simulink model "lab3_ss_srl"  (R2024b)
settings: Solver=ode45  StartTime=0.0  StopTime=sIn.simulation_time  RelTol=1e-3
undefined symbols (not defined in the file or in its folder): daq, drv, feedback, filt, gbox, mld, mot, rads2rpm, sens, sIn
settings Model: Creator=pries  LastModifiedBy=Nihal
settings DataIOCC: SaveOutput=off  SaveTime=off  ReturnWorkspaceOutputs=off

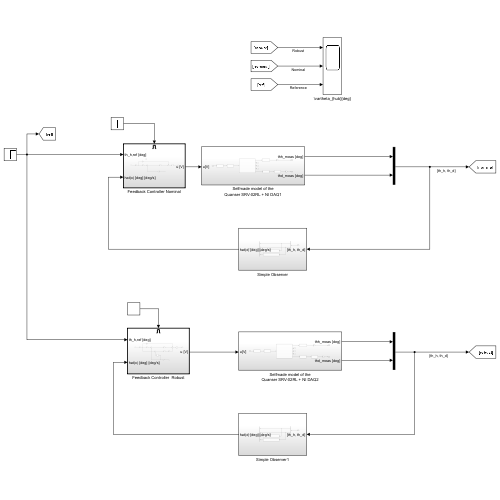
[thumbnail: Simulink's stored preview of the top-level diagram]
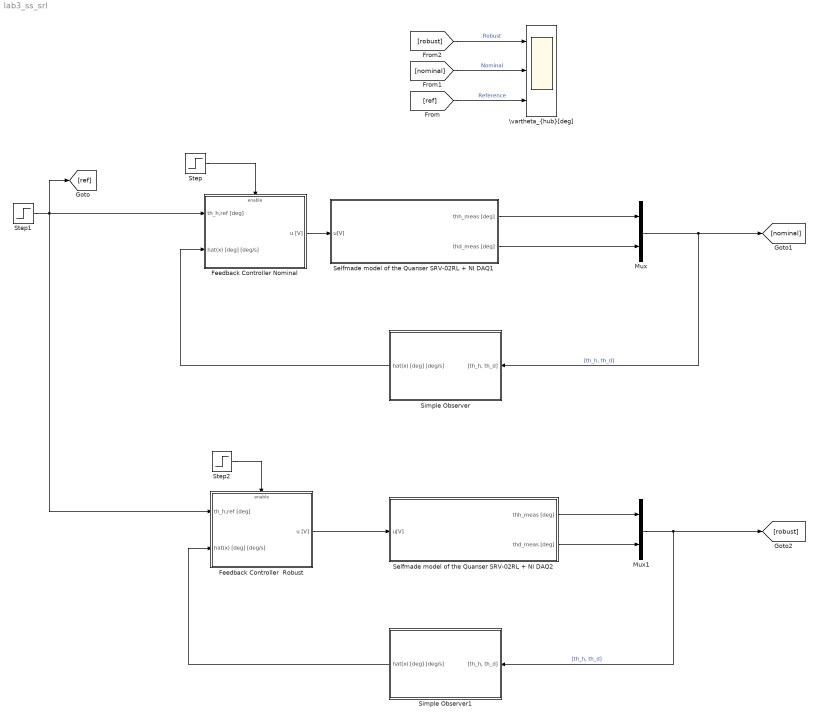
== system lab3_ss_srl ==
  Feedback Controller  Robust : Subsystem
  Feedback Controller Nominal : Subsystem
  Mux : Mux  Inputs=2
  Mux1 : Mux  Inputs=2
  Selfmade model of the Quanser SRV-02RL + NI DAQ1 : Subsystem
  Selfmade model of the Quanser SRV-02RL + NI DAQ2 : Subsystem
  Simple Observer : Subsystem
  Simple Observer1 : Subsystem
  Step : Step  Time=sIn.t1  SampleTime=0
  Step1 : Step  Time=sIn.t1  After=sIn.position  SampleTime=0
  Step2 : Step  Time=sIn.t1  SampleTime=0
  "\\vartheta_{hub}[deg]" : Scope  NumInputPorts=3
  wires:
  Mux/1 -> [nominal], Simple Observer/1("[th_h, th_d]")  "[th_h, th_d]"
  Simple Observer/1(hat(x) [deg] [deg/s]) -> Feedback Controller Nominal/2(hat(x) [deg] [deg/s])
  Step/1 -> Feedback Controller Nominal/Enable
  Step1/1 -> Feedback Controller  Robust/1(th_h,ref [deg]), Feedback Controller Nominal/1(th_h,ref [deg]), [ref]
  Simple Observer1/1(hat(x) [deg] [deg/s]) -> Feedback Controller  Robust/2(hat(x) [deg] [deg/s])
  [robust] -> "\\vartheta_{hub}[deg]"/1  "Robust"
  [nominal] -> "\\vartheta_{hub}[deg]"/2  "Nominal"
  [ref] -> "\\vartheta_{hub}[deg]"/3  "Reference"
  Feedback Controller  Robust/1(u [V]) -> Selfmade model of the Quanser SRV-02RL + NI DAQ2/1(u[V])
  Step2/1 -> Feedback Controller  Robust/Enable
  Feedback Controller Nominal/1(u [V]) -> Selfmade model of the Quanser SRV-02RL + NI DAQ1/1(u[V])
  Selfmade model of the Quanser SRV-02RL + NI DAQ1/1(thh_meas [deg]) -> Mux/1
  Selfmade model of the Quanser SRV-02RL + NI DAQ1/2(thd_meas [deg]) -> Mux/2
  Selfmade model of the Quanser SRV-02RL + NI DAQ2/1(thh_meas [deg]) -> Mux1/1
  Selfmade model of the Quanser SRV-02RL + NI DAQ2/2(thd_meas [deg]) -> Mux1/2
  Mux1/1 -> [robust], Simple Observer1/1("[th_h, th_d]")  "[th_h, th_d]"

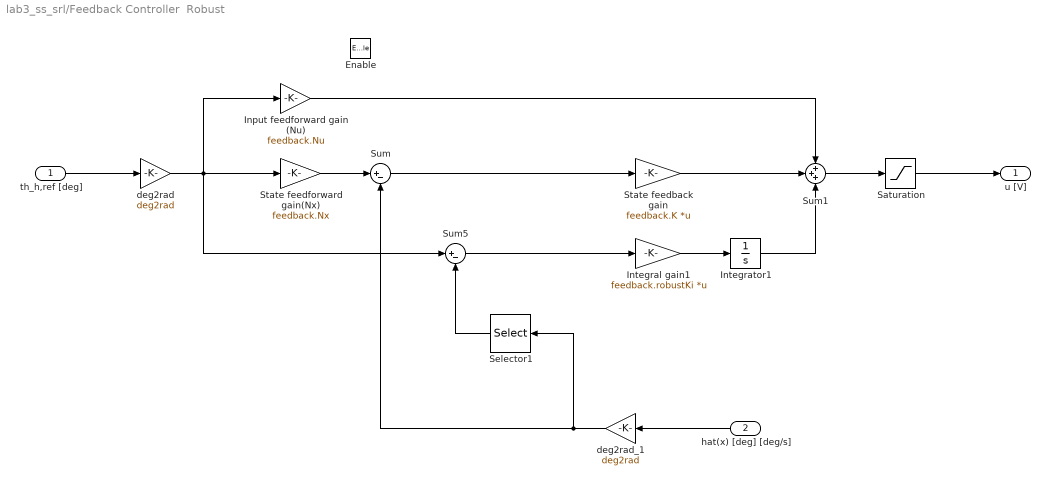
== system lab3_ss_srl/Feedback Controller  Robust ==
  th_h,ref [deg] : Inport
  hat(x) [deg] [deg/s] : Inport  Port=2
  Enable : EnablePort
  Input feedforward gain (Nu) : Gain  Gain=feedback.Nu
  Integral gain1 : Gain  Gain=feedback.robustKi  Multiplication=Matrix(K*u)
  Integrator1 : Integrator
  Saturation : Saturate  UpperLimit=10  LowerLimit=-10
  Selector1 : Selector  InputPortWidth=4  IndexOptions=Index vector (dialog)  Indices=1  OutputSizes=1
  State feedback gain : Gain  Gain=feedback.K  Multiplication=Matrix(K*u)
  State feedforward gain(Nx) : Gain  Gain=feedback.Nx
  Sum : Sum  Inputs=|+-
  Sum1 : Sum  Inputs=+++
  Sum5 : Sum  Inputs=|+-
  deg2rad : Gain  Gain=deg2rad
  deg2rad_1 : Gain  Gain=deg2rad
  u [V] : Outport
  wires:
  Input feedforward gain (Nu)/1 -> Sum1/1
  State feedback gain/1 -> Sum1/2
  Sum1/1 -> Saturation/1
  Sum/1 -> State feedback gain/1
  Saturation/1 -> u [V]/1
  State feedforward gain(Nx)/1 -> Sum/1
  th_h,ref [deg]/1 -> deg2rad/1
  hat(x) [deg] [deg/s]/1 -> deg2rad_1/1
  deg2rad/1 -> Input feedforward gain (Nu)/1, Sum5/1, State feedforward gain(Nx)/1
  Selector1/1 -> Sum5/2
  Integral gain1/1 -> Integrator1/1
  Integrator1/1 -> Sum1/3
  deg2rad_1/1 -> Selector1/1, Sum/2
  Sum5/1 -> Integral gain1/1

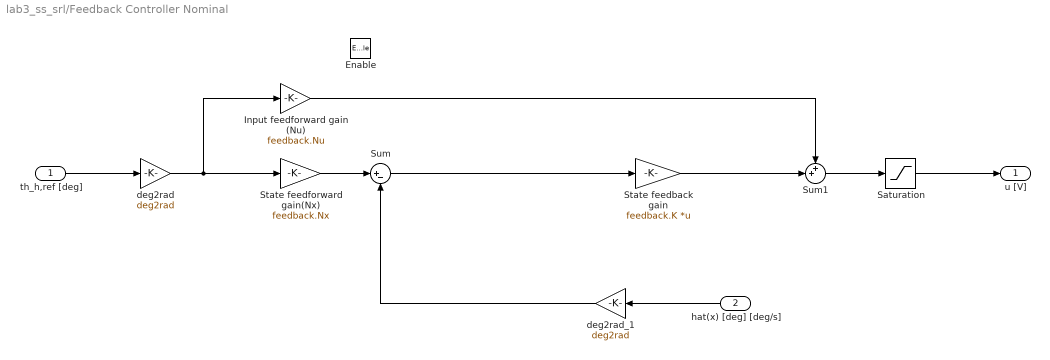
== system lab3_ss_srl/Feedback Controller Nominal ==
  th_h,ref [deg] : Inport
  hat(x) [deg] [deg/s] : Inport  Port=2
  Enable : EnablePort
  Input feedforward gain (Nu) : Gain  Gain=feedback.Nu
  Saturation : Saturate  UpperLimit=10  LowerLimit=-10
  State feedback gain : Gain  Gain=feedback.K  Multiplication=Matrix(K*u)
  State feedforward gain(Nx) : Gain  Gain=feedback.Nx
  Sum : Sum  Inputs=|+-
  Sum1 : Sum  Inputs=++|
  deg2rad : Gain  Gain=deg2rad
  deg2rad_1 : Gain  Gain=deg2rad
  u [V] : Outport
  wires:
  deg2rad_1/1 -> Sum/2
  Input feedforward gain (Nu)/1 -> Sum1/1
  State feedback gain/1 -> Sum1/2
  Sum1/1 -> Saturation/1
  Sum/1 -> State feedback gain/1
  Saturation/1 -> u [V]/1
  State feedforward gain(Nx)/1 -> Sum/1
  deg2rad/1 -> State feedforward gain(Nx)/1, Input feedforward gain (Nu)/1
  th_h,ref [deg]/1 -> deg2rad/1
  hat(x) [deg] [deg/s]/1 -> deg2rad_1/1

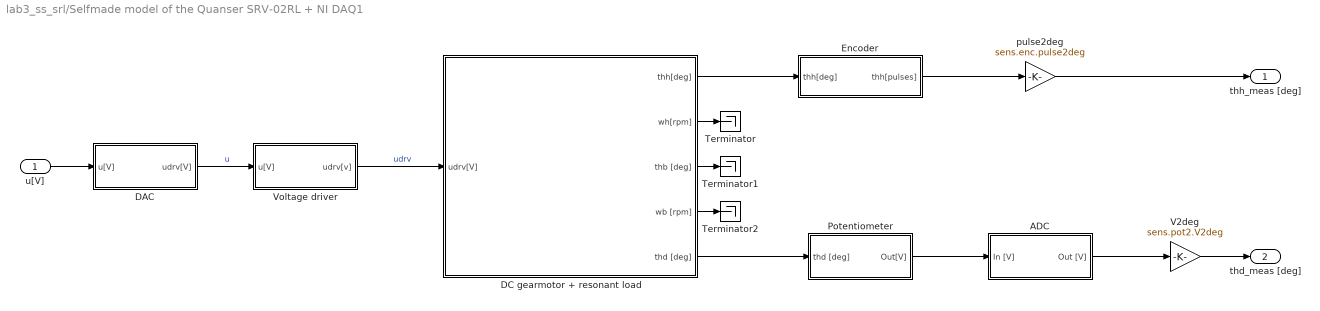
== system lab3_ss_srl/Selfmade model of the Quanser SRV-02RL + NI DAQ1 ==
  u[V] : Inport
  ADC : Subsystem
  DAC : Subsystem
  DC gearmotor + resonant load : Subsystem
  Encoder : Subsystem
  Potentiometer : Subsystem
  Terminator : Terminator
  Terminator1 : Terminator
  Terminator2 : Terminator
  V2deg : Gain  Gain=sens.pot2.V2deg
  Voltage driver : Subsystem
  pulse2deg : Gain  Gain=sens.enc.pulse2deg
  thh_meas [deg] : Outport
  thd_meas [deg] : Outport  Port=2
  wires:
  u[V]/1 -> DAC/1(u[V])
  DAC/1(udrv[V]) -> Voltage driver/1(u[V])  "u"
  Voltage driver/1(udrv[v]) -> DC gearmotor + resonant load/1(udrv[V])  "udrv"
  DC gearmotor + resonant load/1(thh[deg]) -> Encoder/1(thh[deg])
  Encoder/1(thh[pulses]) -> pulse2deg/1
  pulse2deg/1 -> thh_meas [deg]/1
  V2deg/1 -> thd_meas [deg]/1
  DC gearmotor + resonant load/5(thd [deg]) -> Potentiometer/1(thd [deg])
  DC gearmotor + resonant load/4(wb [rpm]) -> Terminator2/1
  DC gearmotor + resonant load/3(thb [deg]) -> Terminator1/1
  DC gearmotor + resonant load/2(wh[rpm]) -> Terminator/1
  Potentiometer/1(Out[V]) -> ADC/1(In [V])
  ADC/1(Out [V]) -> V2deg/1

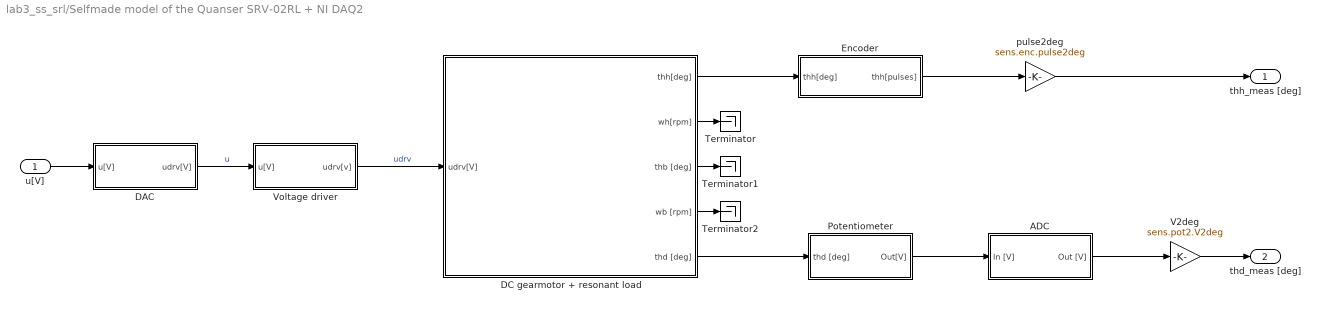
== system lab3_ss_srl/Selfmade model of the Quanser SRV-02RL + NI DAQ2 ==
  u[V] : Inport
  ADC : Subsystem
  DAC : Subsystem
  DC gearmotor + resonant load : Subsystem
  Encoder : Subsystem
  Potentiometer : Subsystem
  Terminator : Terminator
  Terminator1 : Terminator
  Terminator2 : Terminator
  V2deg : Gain  Gain=sens.pot2.V2deg
  Voltage driver : Subsystem
  pulse2deg : Gain  Gain=sens.enc.pulse2deg
  thh_meas [deg] : Outport
  thd_meas [deg] : Outport  Port=2
  wires:
  u[V]/1 -> DAC/1(u[V])
  DAC/1(udrv[V]) -> Voltage driver/1(u[V])  "u"
  Voltage driver/1(udrv[v]) -> DC gearmotor + resonant load/1(udrv[V])  "udrv"
  DC gearmotor + resonant load/1(thh[deg]) -> Encoder/1(thh[deg])
  Encoder/1(thh[pulses]) -> pulse2deg/1
  pulse2deg/1 -> thh_meas [deg]/1
  V2deg/1 -> thd_meas [deg]/1
  DC gearmotor + resonant load/5(thd [deg]) -> Potentiometer/1(thd [deg])
  DC gearmotor + resonant load/4(wb [rpm]) -> Terminator2/1
  DC gearmotor + resonant load/3(thb [deg]) -> Terminator1/1
  DC gearmotor + resonant load/2(wh[rpm]) -> Terminator/1
  Potentiometer/1(Out[V]) -> ADC/1(In [V])
  ADC/1(Out [V]) -> V2deg/1

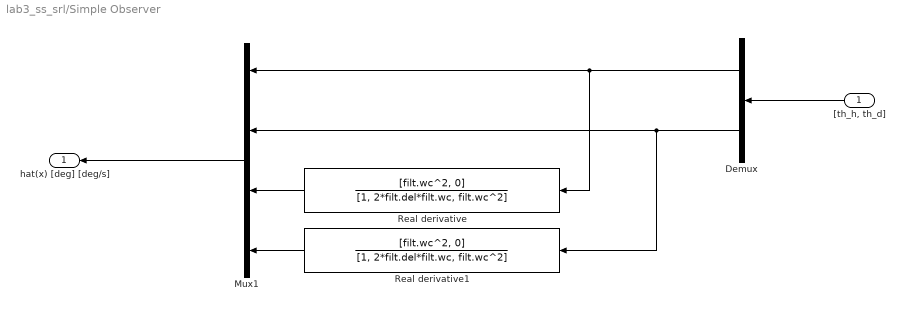
== system lab3_ss_srl/Simple Observer ==
  "[th_h, th_d]" : Inport
  Demux : Demux  Outputs=2
  Mux1 : Mux
  Real derivative : TransferFcn  Numerator=[filt.wc^2, 0]  Denominator=[1, 2*filt.del*filt.wc, filt.wc^2]
  Real derivative1 : TransferFcn  Numerator=[filt.wc^2, 0]  Denominator=[1, 2*filt.del*filt.wc, filt.wc^2]
  hat(x) [deg] [deg/s] : Outport
  wires:
  Demux/1 -> Mux1/1, Real derivative/1
  Mux1/1 -> hat(x) [deg] [deg/s]/1
  "[th_h, th_d]"/1 -> Demux/1
  Real derivative/1 -> Mux1/3
  Demux/2 -> Real derivative1/1, Mux1/2
  Real derivative1/1 -> Mux1/4

== system lab3_ss_srl/Simple Observer1 ==
  "[th_h, th_d]" : Inport
  Demux : Demux  Outputs=2
  Mux1 : Mux
  Real derivative : TransferFcn  Numerator=[filt.wc^2, 0]  Denominator=[1, 2*filt.del*filt.wc, filt.wc^2]
  Real derivative1 : TransferFcn  Numerator=[filt.wc^2, 0]  Denominator=[1, 2*filt.del*filt.wc, filt.wc^2]
  hat(x) [deg] [deg/s] : Outport
  wires:
  Real derivative1/1 -> Mux1/4
  Demux/2 -> Mux1/2, Real derivative1/1
  Real derivative/1 -> Mux1/3
  "[th_h, th_d]"/1 -> Demux/1
  Mux1/1 -> hat(x) [deg] [deg/s]/1
  Demux/1 -> Real derivative/1, Mux1/1

== system lab3_ss_srl/Selfmade model of the Quanser SRV-02RL + NI DAQ1/ADC ==
  In [V] : Inport
  ADC Sampling : ZeroOrderHold  SampleTime=daq.adc.Ts
  ADC Saturation : Saturate  UpperLimit=2.5  LowerLimit=-2.5
  ADC quantization : Quantizer  QuantizationInterval=daq.adc.q
  Out [V] : Outport
  wires:
  In [V]/1 -> ADC Sampling/1
  ADC Sampling/1 -> ADC quantization/1
  ADC quantization/1 -> ADC Saturation/1
  ADC Saturation/1 -> Out [V]/1

== system lab3_ss_srl/Selfmade model of the Quanser SRV-02RL + NI DAQ1/DAC ==
  u[V] : Inport
  Quantizer : Quantizer  QuantizationInterval=daq.dac.q
  Saturation : Saturate  UpperLimit=10  LowerLimit=-10
  Zero-Order Hold : ZeroOrderHold  SampleTime=1e-3
  udrv[V] : Outport
  wires:
  Zero-Order Hold/1 -> Quantizer/1
  u[V]/1 -> Zero-Order Hold/1
  Quantizer/1 -> Saturation/1
  Saturation/1 -> udrv[V]/1

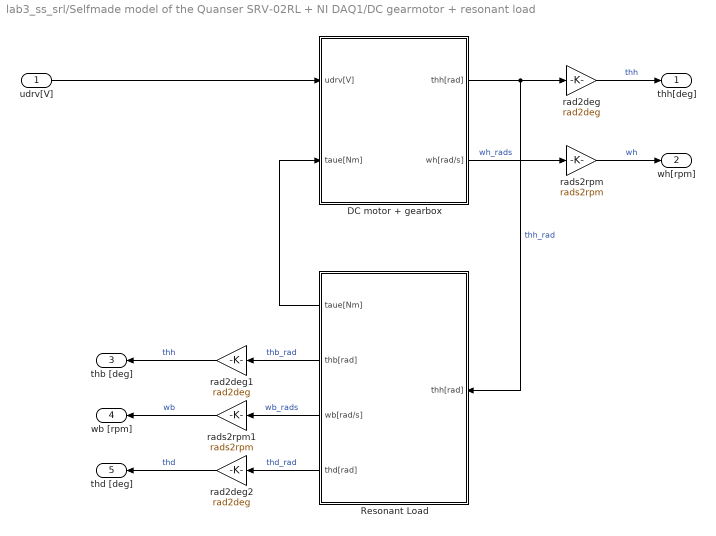
== system lab3_ss_srl/Selfmade model of the Quanser SRV-02RL + NI DAQ1/DC gearmotor + resonant load ==
  udrv[V] : Inport
  DC motor + gearbox : Subsystem
  Resonant Load : Subsystem
  rad2deg : Gain  Gain=rad2deg
  rad2deg1 : Gain  Gain=rad2deg
  rad2deg2 : Gain  Gain=rad2deg
  rads2rpm : Gain  Gain=rads2rpm
  rads2rpm1 : Gain  Gain=rads2rpm
  thh[deg] : Outport
  wh[rpm] : Outport  Port=2
  thb [deg] : Outport  Port=3
  wb [rpm] : Outport  Port=4
  thd [deg] : Outport  Port=5
  wires:
  DC motor + gearbox/1(thh[rad]) -> Resonant Load/1(thh[rad]), rad2deg/1  "thh_rad"
  Resonant Load/2(thb[rad]) -> rad2deg1/1  "thb_rad"
  rad2deg2/1 -> thd [deg]/1  "thd"
  rad2deg/1 -> thh[deg]/1  "thh"
  Resonant Load/4(thd[rad]) -> rad2deg2/1  "thd_rad"
  Resonant Load/1(taue[Nm]) -> DC motor + gearbox/2(taue[Nm])
  rad2deg1/1 -> thb [deg]/1  "thh"
  rads2rpm1/1 -> wb [rpm]/1  "wb"
  Resonant Load/3(wb[rad/s]) -> rads2rpm1/1  "wb_rads"
  DC motor + gearbox/2(wh[rad/s]) -> rads2rpm/1  "wh_rads"
  rads2rpm/1 -> wh[rpm]/1  "wh"
  udrv[V]/1 -> DC motor + gearbox/1(udrv[V])

== system lab3_ss_srl/Selfmade model of the Quanser SRV-02RL + NI DAQ1/Encoder ==
  thh[deg] : Inport
  Gain : Gain  Gain=1/sens.enc.pulse2deg
  Quantizer : Quantizer  QuantizationInterval=sens.enc.pulse2deg
  Zero-Order Hold : ZeroOrderHold  SampleTime=1e-3
  thh[pulses] : Outport
  wires:
  thh[deg]/1 -> Zero-Order Hold/1
  Gain/1 -> thh[pulses]/1
  Quantizer/1 -> Gain/1
  Zero-Order Hold/1 -> Quantizer/1

== system lab3_ss_srl/Selfmade model of the Quanser SRV-02RL + NI DAQ1/Potentiometer ==
  thd [deg] : Inport
  Sensor output noise [V] : RandomNumber  Variance=sens.pot2.noise.var  SampleTime=daq.adc.Ts
  Sum : Sum  Inputs=|++
  deg2V : Gain  Gain=sens.pot2.deg2V
  Out[V] : Outport
  wires:
  thd [deg]/1 -> deg2V/1
  deg2V/1 -> Sum/1
  Sensor output noise [V]/1 -> Sum/2
  Sum/1 -> Out[V]/1

== system lab3_ss_srl/Selfmade model of the Quanser SRV-02RL + NI DAQ1/Voltage driver ==
  u[V] : Inport
  Saturation : Saturate  UpperLimit=12  LowerLimit=-12
  Transfer Fcn : TransferFcn  Numerator=[drv.dcgain]  Denominator=[drv.Tc 1]
  udrv[v] : Outport
  wires:
  u[V]/1 -> Transfer Fcn/1
  Transfer Fcn/1 -> Saturation/1
  Saturation/1 -> udrv[v]/1

== system lab3_ss_srl/Selfmade model of the Quanser SRV-02RL + NI DAQ2/ADC ==
  In [V] : Inport
  ADC Sampling : ZeroOrderHold  SampleTime=daq.adc.Ts
  ADC Saturation : Saturate  UpperLimit=2.5  LowerLimit=-2.5
  ADC quantization : Quantizer  QuantizationInterval=daq.adc.q
  Out [V] : Outport
  wires:
  In [V]/1 -> ADC Sampling/1
  ADC Sampling/1 -> ADC quantization/1
  ADC quantization/1 -> ADC Saturation/1
  ADC Saturation/1 -> Out [V]/1

== system lab3_ss_srl/Selfmade model of the Quanser SRV-02RL + NI DAQ2/DAC ==
  u[V] : Inport
  Quantizer : Quantizer  QuantizationInterval=daq.dac.q
  Saturation : Saturate  UpperLimit=10  LowerLimit=-10
  Zero-Order Hold : ZeroOrderHold  SampleTime=1e-3
  udrv[V] : Outport
  wires:
  Zero-Order Hold/1 -> Quantizer/1
  u[V]/1 -> Zero-Order Hold/1
  Quantizer/1 -> Saturation/1
  Saturation/1 -> udrv[V]/1

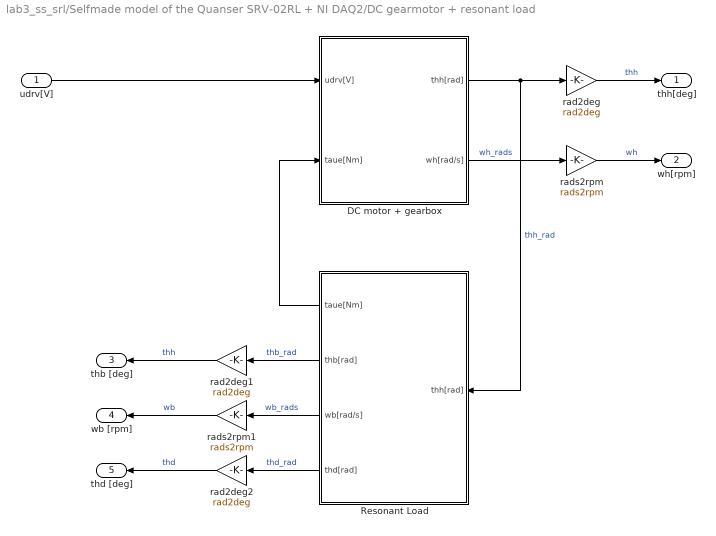
== system lab3_ss_srl/Selfmade model of the Quanser SRV-02RL + NI DAQ2/DC gearmotor + resonant load ==
  udrv[V] : Inport
  DC motor + gearbox : Subsystem
  Resonant Load : Subsystem
  rad2deg : Gain  Gain=rad2deg
  rad2deg1 : Gain  Gain=rad2deg
  rad2deg2 : Gain  Gain=rad2deg
  rads2rpm : Gain  Gain=rads2rpm
  rads2rpm1 : Gain  Gain=rads2rpm
  thh[deg] : Outport
  wh[rpm] : Outport  Port=2
  thb [deg] : Outport  Port=3
  wb [rpm] : Outport  Port=4
  thd [deg] : Outport  Port=5
  wires:
  DC motor + gearbox/1(thh[rad]) -> Resonant Load/1(thh[rad]), rad2deg/1  "thh_rad"
  Resonant Load/2(thb[rad]) -> rad2deg1/1  "thb_rad"
  rad2deg2/1 -> thd [deg]/1  "thd"
  rad2deg/1 -> thh[deg]/1  "thh"
  Resonant Load/4(thd[rad]) -> rad2deg2/1  "thd_rad"
  Resonant Load/1(taue[Nm]) -> DC motor + gearbox/2(taue[Nm])
  rad2deg1/1 -> thb [deg]/1  "thh"
  rads2rpm1/1 -> wb [rpm]/1  "wb"
  Resonant Load/3(wb[rad/s]) -> rads2rpm1/1  "wb_rads"
  DC motor + gearbox/2(wh[rad/s]) -> rads2rpm/1  "wh_rads"
  rads2rpm/1 -> wh[rpm]/1  "wh"
  udrv[V]/1 -> DC motor + gearbox/1(udrv[V])

== system lab3_ss_srl/Selfmade model of the Quanser SRV-02RL + NI DAQ2/Encoder ==
  thh[deg] : Inport
  Gain : Gain  Gain=1/sens.enc.pulse2deg
  Quantizer : Quantizer  QuantizationInterval=sens.enc.pulse2deg
  Zero-Order Hold : ZeroOrderHold  SampleTime=1e-3
  thh[pulses] : Outport
  wires:
  thh[deg]/1 -> Zero-Order Hold/1
  Gain/1 -> thh[pulses]/1
  Quantizer/1 -> Gain/1
  Zero-Order Hold/1 -> Quantizer/1

== system lab3_ss_srl/Selfmade model of the Quanser SRV-02RL + NI DAQ2/Potentiometer ==
  thd [deg] : Inport
  Sensor output noise [V] : RandomNumber  Variance=sens.pot2.noise.var  SampleTime=daq.adc.Ts
  Sum : Sum  Inputs=|++
  deg2V : Gain  Gain=sens.pot2.deg2V
  Out[V] : Outport
  wires:
  thd [deg]/1 -> deg2V/1
  deg2V/1 -> Sum/1
  Sensor output noise [V]/1 -> Sum/2
  Sum/1 -> Out[V]/1

== system lab3_ss_srl/Selfmade model of the Quanser SRV-02RL + NI DAQ2/Voltage driver ==
  u[V] : Inport
  Saturation : Saturate  UpperLimit=12  LowerLimit=-12
  Transfer Fcn : TransferFcn  Numerator=[drv.dcgain]  Denominator=[drv.Tc 1]
  udrv[v] : Outport
  wires:
  u[V]/1 -> Transfer Fcn/1
  Transfer Fcn/1 -> Saturation/1
  Saturation/1 -> udrv[v]/1

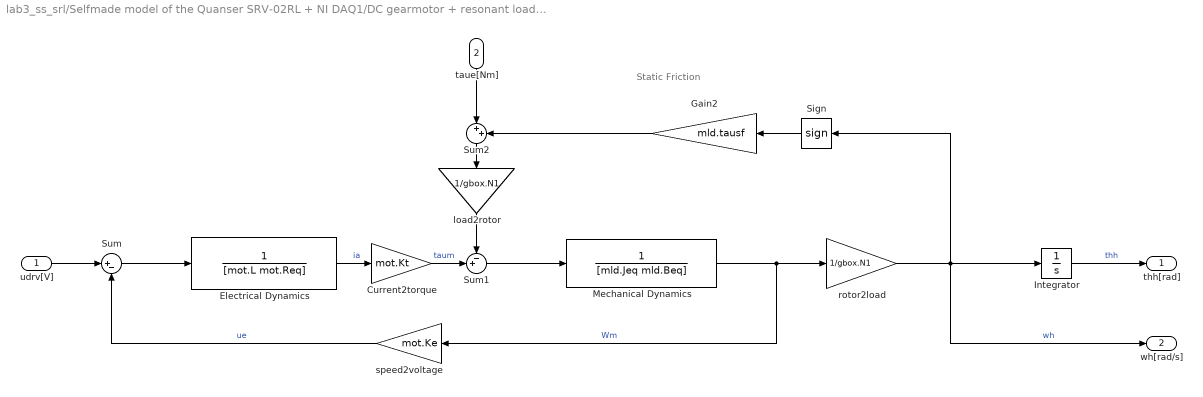
== system lab3_ss_srl/Selfmade model of the Quanser SRV-02RL + NI DAQ1/DC gearmotor + resonant load/DC motor + gearbox ==
  note: Static Friction
  udrv[V] : Inport
  taue[Nm] : Inport  Port=2
  Current2torque : Gain  Gain=mot.Kt
  Electrical Dynamics : TransferFcn  Denominator=[mot.L mot.Req]
  Gain2 : Gain  Gain=mld.tausf
  Integrator : Integrator
  Mechanical Dynamics : TransferFcn  Denominator=[mld.Jeq mld.Beq]
  Sign : Signum  ZeroCross=off
  Sum : Sum  Inputs=|+-
  Sum1 : Sum  Inputs=-+|
  Sum2 : Sum  Inputs=|++
  load2rotor : Gain  Gain=1/gbox.N1
  rotor2load : Gain  Gain=1/gbox.N1
  speed2voltage : Gain  Gain=mot.Ke
  thh[rad] : Outport
  wh[rad/s] : Outport  Port=2
  wires:
  udrv[V]/1 -> Sum/1
  Sum/1 -> Electrical Dynamics/1
  Electrical Dynamics/1 -> Current2torque/1  "ia"
  load2rotor/1 -> Sum1/1
  Sign/1 -> Gain2/1
  Mechanical Dynamics/1 -> speed2voltage/1, rotor2load/1  "Wm"
  rotor2load/1 -> wh[rad/s]/1, Sign/1, Integrator/1  "wh"
  Sum1/1 -> Mechanical Dynamics/1
  Current2torque/1 -> Sum1/2  "taum"
  speed2voltage/1 -> Sum/2  "ue"
  Integrator/1 -> thh[rad]/1  "thh"
  taue[Nm]/1 -> Sum2/1
  Sum2/1 -> load2rotor/1
  Gain2/1 -> Sum2/2

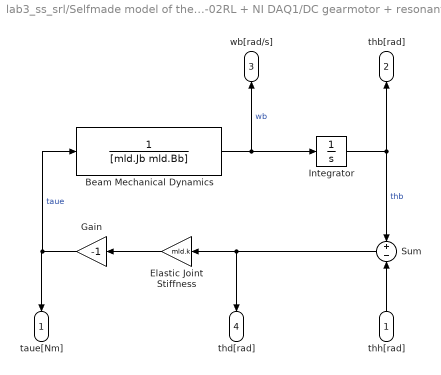
== system lab3_ss_srl/Selfmade model of the Quanser SRV-02RL + NI DAQ1/DC gearmotor + resonant load/Resonant Load ==
  thh[rad] : Inport
  Beam Mechanical Dynamics : TransferFcn  Denominator=[mld.Jb mld.Bb]
  Elastic Joint Stiffness : Gain  Gain=mld.k
  Gain : Gain  Gain=-1
  Integrator : Integrator
  Sum : Sum  Inputs=+|-
  taue[Nm] : Outport
  thb[rad] : Outport  Port=2
  wb[rad/s] : Outport  Port=3
  thd[rad] : Outport  Port=4
  wires:
  thh[rad]/1 -> Sum/2
  Integrator/1 -> Sum/1, thb[rad]/1  "thb"
  Sum/1 -> thd[rad]/1, Elastic Joint Stiffness/1
  Elastic Joint Stiffness/1 -> Gain/1
  Gain/1 -> Beam Mechanical Dynamics/1, taue[Nm]/1  "taue"
  Beam Mechanical Dynamics/1 -> wb[rad/s]/1, Integrator/1  "wb"

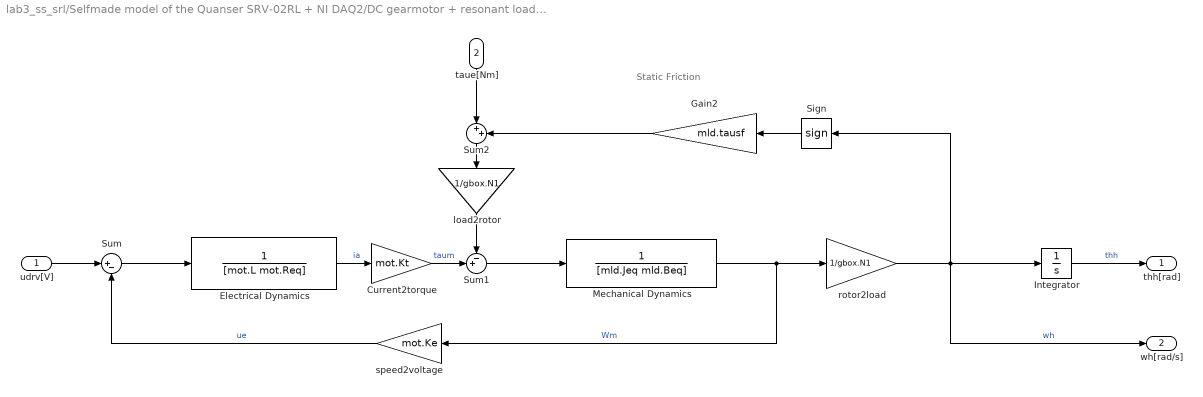
== system lab3_ss_srl/Selfmade model of the Quanser SRV-02RL + NI DAQ2/DC gearmotor + resonant load/DC motor + gearbox ==
  note: Static Friction
  udrv[V] : Inport
  taue[Nm] : Inport  Port=2
  Current2torque : Gain  Gain=mot.Kt
  Electrical Dynamics : TransferFcn  Denominator=[mot.L mot.Req]
  Gain2 : Gain  Gain=mld.tausf
  Integrator : Integrator
  Mechanical Dynamics : TransferFcn  Denominator=[mld.Jeq mld.Beq]
  Sign : Signum  ZeroCross=off
  Sum : Sum  Inputs=|+-
  Sum1 : Sum  Inputs=-+|
  Sum2 : Sum  Inputs=|++
  load2rotor : Gain  Gain=1/gbox.N1
  rotor2load : Gain  Gain=1/gbox.N1
  speed2voltage : Gain  Gain=mot.Ke
  thh[rad] : Outport
  wh[rad/s] : Outport  Port=2
  wires:
  udrv[V]/1 -> Sum/1
  Sum/1 -> Electrical Dynamics/1
  Electrical Dynamics/1 -> Current2torque/1  "ia"
  load2rotor/1 -> Sum1/1
  Sign/1 -> Gain2/1
  Mechanical Dynamics/1 -> speed2voltage/1, rotor2load/1  "Wm"
  rotor2load/1 -> wh[rad/s]/1, Sign/1, Integrator/1  "wh"
  Sum1/1 -> Mechanical Dynamics/1
  Current2torque/1 -> Sum1/2  "taum"
  speed2voltage/1 -> Sum/2  "ue"
  Integrator/1 -> thh[rad]/1  "thh"
  taue[Nm]/1 -> Sum2/1
  Sum2/1 -> load2rotor/1
  Gain2/1 -> Sum2/2

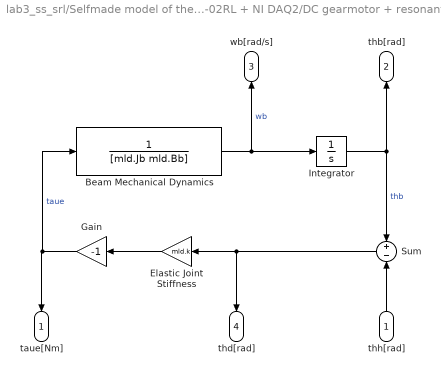
== system lab3_ss_srl/Selfmade model of the Quanser SRV-02RL + NI DAQ2/DC gearmotor + resonant load/Resonant Load ==
  thh[rad] : Inport
  Beam Mechanical Dynamics : TransferFcn  Denominator=[mld.Jb mld.Bb]
  Elastic Joint Stiffness : Gain  Gain=mld.k
  Gain : Gain  Gain=-1
  Integrator : Integrator
  Sum : Sum  Inputs=+|-
  taue[Nm] : Outport
  thb[rad] : Outport  Port=2
  wb[rad/s] : Outport  Port=3
  thd[rad] : Outport  Port=4
  wires:
  thh[rad]/1 -> Sum/2
  Integrator/1 -> Sum/1, thb[rad]/1  "thb"
  Sum/1 -> thd[rad]/1, Elastic Joint Stiffness/1
  Elastic Joint Stiffness/1 -> Gain/1
  Gain/1 -> Beam Mechanical Dynamics/1, taue[Nm]/1  "taue"
  Beam Mechanical Dynamics/1 -> wb[rad/s]/1, Integrator/1  "wb"
